simulink model "Trabajo_final_FSK"  (R2023b)
settings: Solver=FixedStepDiscrete  StartTime=0.0  StopTime=263  RelTol=1e-3
libraries: commdigbbndfm2 x2, commchan3 x1
settings Model: Creator=Enmanel Toribio  LastModifiedBy=Enmanel Toribio

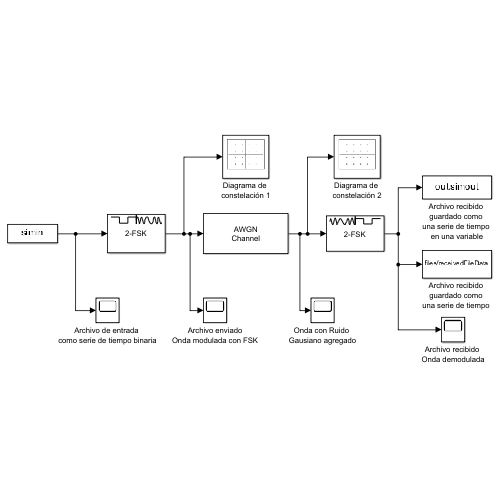
[thumbnail: Simulink's stored preview of the top-level diagram]
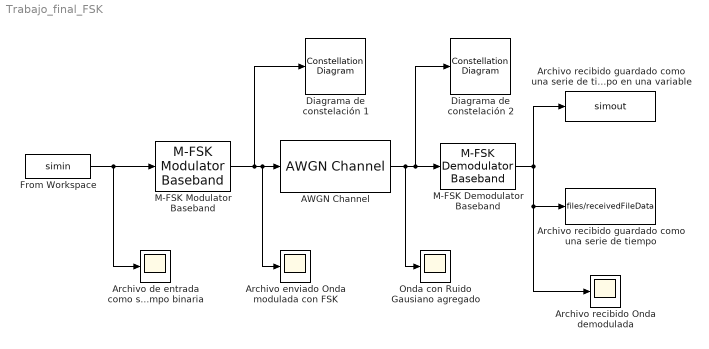
== system Trabajo_final_FSK ==
  AWGN Channel : commchan3/AWGN Channel  LegacyMode=off  NoiseMethod="Signal to noise ratio  (SNR)"  noiseMode="Signal to noise ratio  (SNR)"  EbNo=10  EsNo=10  SNR=20  BitsPerSymbol=1  SignalPower=1  SamplesPerSymbol=1  SymbolPeriod=1  VarianceSource=Parameter  Variance=1  RandomStream=Global stream  Seed=67  SimulateUsing=Code generation
  Archivo de entrada como serie de tiempo binaria : Scope
  Archivo enviado Onda modulada con FSK : Scope
  Archivo recibido Onda demodulada : Scope
  "Archivo recibido guardado como una serie de tiempo " : ToFile  Filename=files/receivedFileData  MatrixName=received_file_data  SampleTime=1
  Archivo recibido guardado como una serie de tiempo en una variable : ToWorkspace  VariableName=simout  SaveFormat=Timeseries  SampleTime=1
  Diagrama de constelación 1 : ConstellationDiagram  WindowPosition=[-1356.000000,305.000000,600.000000,521.000000,]  ScopeFrameLocation=window  DefaultConfigurationName=comm.scopes.ConstellationDiagramBlockCfg
  Diagrama de constelación 2 : ConstellationDiagram  WindowPosition=[-696.000000,272.000000,600.000000,600.000000,]  ScopeFrameLocation=window  DefaultConfigurationName=comm.scopes.ConstellationDiagramBlockCfg
  From Workspace : FromWorkspace  VariableName=simin  SampleTime=1
  M-FSK Demodulator Baseband : commdigbbndfm2/M-FSK Demodulator Baseband  M=2  OutType=Integer  Dec=Gray  freqSep=100  numSamp=8  RateOptions=Enforce single-rate processing  outDataType=double
  M-FSK Modulator Baseband : commdigbbndfm2/M-FSK Modulator Baseband  M=2  InType=Integer  Enc=Gray  freqSep=100  phaseType=Continuous  numSamp=8  RateOptions=Enforce single-rate processing  outDataType=single
  Onda con Ruido Gausiano agregado : Scope
  wires:
  From Workspace/1 -> Archivo de entrada como serie de tiempo binaria/1, M-FSK Modulator Baseband/1
  AWGN Channel/1 -> Onda con Ruido Gausiano agregado/1, Diagrama de constelación 2/1, M-FSK Demodulator Baseband/1
  M-FSK Demodulator Baseband/1 -> "Archivo recibido guardado como una serie de tiempo "/1, Archivo recibido Onda demodulada/1, Archivo recibido guardado como una serie de tiempo en una variable/1
  M-FSK Modulator Baseband/1 -> Diagrama de constelación 1/1, Archivo enviado Onda modulada con FSK/1, AWGN Channel/1
